simulink library "Lib_PF_LineDC_TMATS"  (R2017a)
settings: Solver=ode45  StartTime=0.0  StopTime=10.0  RelTol=1e-3  EnableMultiTasking=on
Description:
  | Thomas Modules
settings Model: Creator=jwchapm2  LastModifiedBy=glthoma1
settings DataIOCC: LimitDataPoints=on  SaveFormat=Array
settings OptimizationCC: ExpressionDepthLimit=2147483647  LifeSpan=inf
settings DebuggingCC: UnderspecifiedInitializationDetection=Classic  MergeDetectMultiDrivingBlocksExec=none  SolverPrmCheckMsg=warning  StateNameClashWarn=warning  SFUnexpectedBacktrackingDiag=warning  SFNoUnconditionalDefaultTransitionDiag=warning  SFExecutionAtInitializationDiag=none
settings HardwareCC: ProdBitPerPointer=32  ProdBitPerSizeT=32  ProdBitPerPtrDiffT=32  ProdLargestAtomicFloat=None  ProdIntDivRoundTo=Undefined  ProdEndianess=Unspecified  ProdWordSize=32  ProdHWDeviceType=32-bit Generic
settings ModelReferenceCC: PropagateSignalLabelsOutOfModel=off
settings GRTTargetCC: TargetLangStandard=C89/C90 (ANSI)  GeneratePreprocessorConditionals=Disable all
settings ConfigComp: CovMetricSettings=dw  CovHtmlReporting=on  CovSaveCumulativeToWorkspaceVar=on  CovSaveSingleToWorkspaceVar=on  CovExternalEMLEnable=off

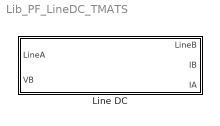
== system Lib_PF_LineDC_TMATS ==
  Line DC : Subsystem  mask{R_M=100}
      mask prompts: R_M "R_M - Z Resistance"
      mask Display:
      | fprintf('R: %g',R_M)
      | port_label('input',1,'VA')
      | port_label('input',2,'VBg')
      | port_label('output',1,'VB')
      | port_label('output',2,'IB')
      | port_label('output',3,'IA')

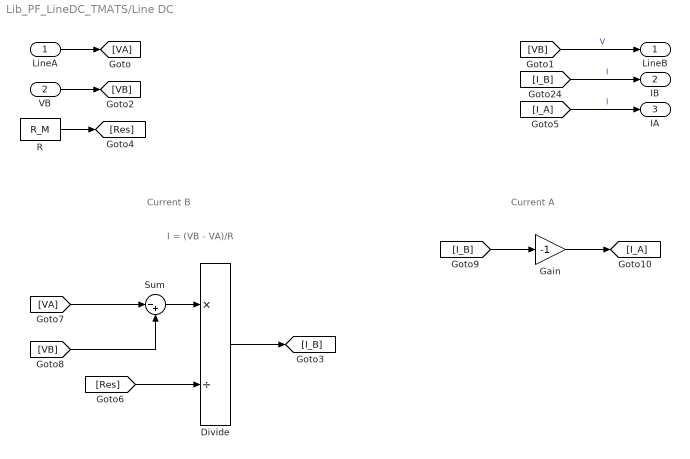
== system Lib_PF_LineDC_TMATS/Line DC ==
  note: I = (VB - VA)/R
  note: Current B
  note: Current A
  LineA : Inport
  VB : Inport  Port=2
  Divide : Product  Inputs=*/
  Gain : Gain  Gain=-1
  R : Constant  Value=R_M
  Sum : Sum  Inputs=|-+
  LineB : Outport
  IB : Outport  Port=2
  IA : Outport  Port=3
  wires:
  LineA/1 -> [VA]
  [I_A] -> IA/1  "I"
  VB/1 -> [VB]
  [VB] -> LineB/1  "V"
  R/1 -> [Res]
  [I_B] -> IB/1  "I"
  [VB] -> Sum/2
  [VA] -> Sum/1
  Divide/1 -> [I_B]
  Sum/1 -> Divide/1
  [Res] -> Divide/2
  [I_B] -> Gain/1
  Gain/1 -> [I_A]
